simulink model "sphereMPC"  (R2020b)
settings: Solver=ode4  StartTime=0  StopTime=400  FixedStep=0.01  MaxStep=0.01  RelTol=1e-3  EnableMultiTasking=on
values from neighbouring files (symbols this model uses):
  simu = simulationClass()    [plotFreqDep.m]    (also in wecSimInputFile.m)
undefined symbols (not defined in the file or in its folder): body, controller, geometry, hydroData, pto
libraries: WECSim_Lib_Frames x1, WECSim_Lib_Body_Elements x1, simulink x1, WECSim_Lib_PTOs x1
settings Model: Creator=mlawson  LastModifiedBy=akeeste
settings SolverCC: ZeroCrossControl=DisableAll  AlgebraicLoopSolver=LineSearch  AutoInsertRateTranBlk=on
settings DataIOCC: SaveFormat=Array  SaveOutput=off  SaveTime=off  ReturnWorkspaceOutputs=off
settings OptimizationCC: LifeSpan=inf  SimCompilerOptimization=on
settings DebuggingCC: MergeDetectMultiDrivingBlocksExec=none  SolverPrmCheckMsg=warning  AllowSymbolicDim=off  StateNameClashWarn=warning  SFUnexpectedBacktrackingDiag=warning  SFNoUnconditionalDefaultTransitionDiag=warning  SFExecutionAtInitializationDiag=none  ArithmeticOperatorsInVariantConditions=warning
settings HardwareCC: ProdBitPerPointer=32  ProdBitPerSizeT=32  ProdBitPerPtrDiffT=32  ProdLargestAtomicFloat=None  ProdIntDivRoundTo=Undefined  ProdEndianess=Unspecified  ProdWordSize=32  ProdHWDeviceType=32-bit Generic
settings ModelReferenceCC: PropagateVarSize=Only when enabling  PropagateSignalLabelsOutOfModel=off
settings SFSimCC: SimUseLocalCustomCode=off  CustomCodeUndefinedFunction=UseInterfaceOnly
settings RTWCC: RTWUseLocalCustomCode=off
settings CodeAppCC: StateflowObjectComments=on
settings GRTTargetCC: TargetLangStandard=C89/C90 (ANSI)
settings ConfigComp: CovMetricSettings=dw  CovSaveCumulativeToWorkspaceVar=on  CovSaveSingleToWorkspaceVar=on  CovExternalEMLEnable=off  CovSFcnEnable=off
settings SimscapeCC: SimscapeNormalizeSystem=off
settings ConfigurationSet: Description=SimMechanics 2G
settings ExplorerConfigSet: InternalSimMechanicsExplorerSettings="<ExplorerConfiguration><canonicalview>default</canonicalview><TilePanel><TileInfo><Tiles Columns=\"1\" Count=\"1\" Rows=\"1\"><Column Left=\"2\" Weight=\"1\"/><Column Left=\"1335\"/><Row Top=\"2\" Weight=\"1\"/><Row Top=\"911\"/><Tile Height=\"1\" Width=\"1\" X=\"0\" Y=\"0\"/></Tiles></TileInfo><SceneInfo><SceneViewer><BGColor><R>0.60000002384185791</R><G>0.60000002384185791</G><B>0.60000002384185791</B></BGColor><Camera><Position><X>365.37645888990272</X><Y>-369.82486814446582</Y><Z>359.64809521743916</Z></Position><Center><X>-6.7351450971904585</X><Y>2.2867358426280204</Y><Z>-12.463508769654169</Z></Center><Up><X>-0.40824829046386307</X><Y>0.40824829046386307</Y><Z>0.81649658092772615</Z></Up><Left>-57.820127362122818</Left><Right>57.820127362122818</Right><Bottom>-38.308817187253304</Bottom><Top>38.308817187253304</Top></Camera></SceneViewer></SceneInfo></TilePanel></ExplorerConfiguration>"

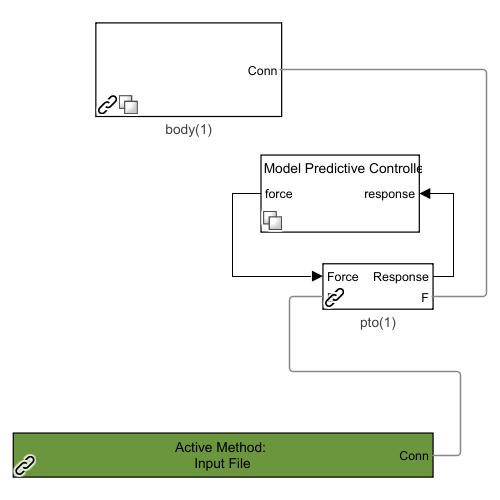
[thumbnail: Simulink's stored preview of the top-level diagram]
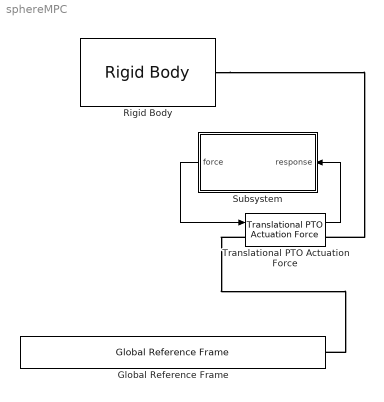
== system sphereMPC ==
  Global Reference Frame : WECSim_Lib_Frames/Global Reference Frame  waves=waves  simu=simu  InputMethod=Input File  InputFile=wecSimInputFile.m  mode=normal  explorer=off  solver=ode4  startTime=0  rampTime=100  endTime=400  dt=0.1  cicEndTime=60  stateSpace=0  WaveClass=regular  height=2.5  period=8  elevationFile=NOT DEFINED  spectrumFile=NOT DEFINED  direction=0  spread=1  spectrumType=NOT DEFINED  phaseSeed=0  option=EqualEnergy
  Rigid Body : WECSim_Lib_Body_Elements/Rigid Body  body=body(1)  h5File=hydroData/*.h5  geometryFile=geometry/*.stl  mass=0  inertia=0 0 0  inertiaProducts=0 0 0  nonHydro=0  nonlinearHydro=0  centerGravity=0 0 0  centerBuoyancy=0 0 0  dof=6  volume=0  QTFs=0  displacement=0 0 0  axis=0 1 0  angle=0  option=0  cd=0 0 0  ca=0 0 0  area=0 0 0  VME=0  rgME=0 0 0  z=0 0 1
  Subsystem : Subsystem  Variant=on  VariantControl=Choice
  Translational PTO Actuation Force : WECSim_Lib_PTOs/Translational PTO Actuation Force  pto=pto(1)  loc="0  0  0"  stiffness=0  damping=0  equilibriumPosition=0  pretension=0  displacement=0 0 0  y=0 1 0  z=0 0 1  upperLimitSpecify=off  upperLimitBound=0  upperLimitTransitionRegionWidth=0  upperLimitStiffness=0  upperLimitDamping=0  lowerLimitSpecify=off  lowerLimitBound=0  lowerLimitTransitionRegionWidth=0  lowerLimitStiffness=0  lowerLimitDamping=0
      settings: AttributesFormatString=%<pto>
  wires:
  Translational PTO Actuation Force/1 -> Subsystem/1(response)
  Subsystem/1(force) -> Translational PTO Actuation Force/1
  connections:
  Rigid Body/RConn1 -- Translational PTO Actuation Force/RConn1
  Translational PTO Actuation Force/LConn1 -- Global Reference Frame/RConn1

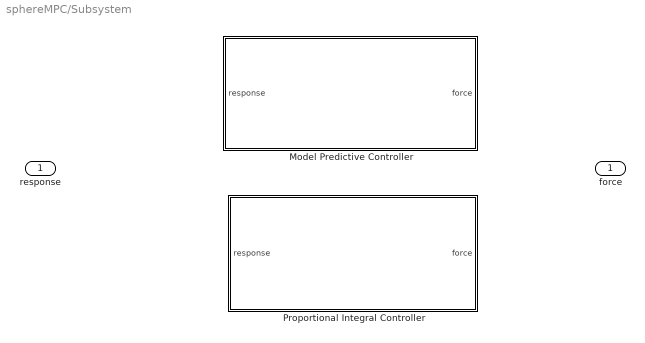
== system sphereMPC/Subsystem ==
  response : Inport
  Model Predictive Controller : Subsystem  VariantControl=controller.MPC == 1
  Proportional Integral Controller : Subsystem  VariantControl=controller.MPC == 0
  force : Outport

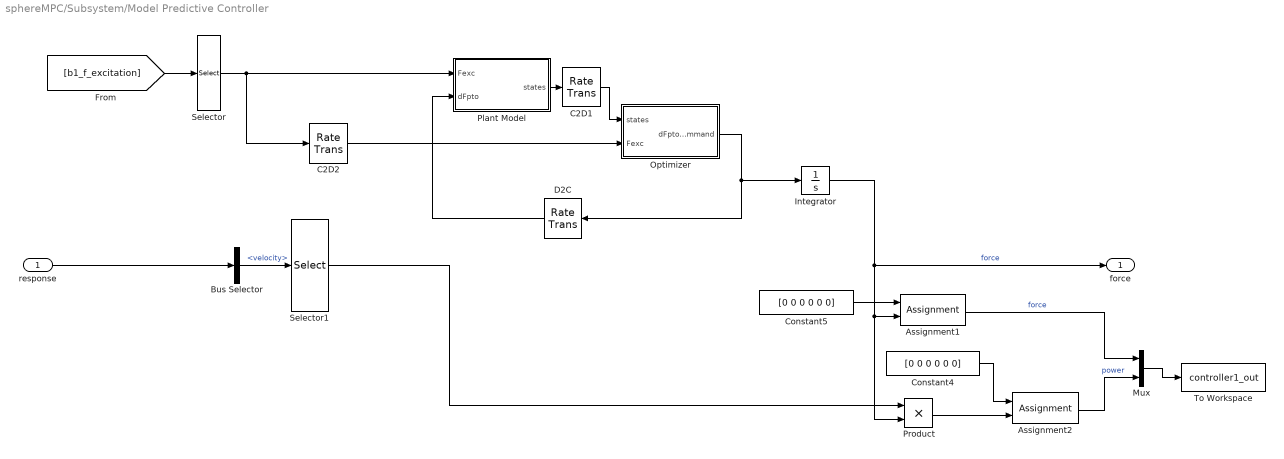
== system sphereMPC/Subsystem/Model Predictive Controller ==
  response : Inport
  Assignment1 : Assignment  IndexOptions=Index vector (dialog)  Indices=3  OutputSizes=1
  Assignment2 : Assignment  IndexOptions=Index vector (dialog)  Indices=3  OutputSizes=1
  Bus Selector : BusSelector  OutputSignals=velocity
  C2D1 : RateTransition  OutPortSampleTime=controller(1).modelPredictiveControl.dt
  C2D2 : RateTransition  OutPortSampleTime=controller(1).modelPredictiveControl.dt
  Constant4 : Constant  Value=[0 0 0 0 0 0]
  Constant5 : Constant  Value=[0 0 0 0 0 0]
  D2C : RateTransition  OutPortSampleTime=simu.dt
  Integrator : Integrator
  Mux : Mux  Inputs=2
  Optimizer : Subsystem
  Plant Model : Subsystem
  Product : Product
  Selector : Selector  InputPortWidth=6  IndexOptions=Index vector (dialog)  Indices=3  OutputSizes=1
  Selector1 : Selector  InputPortWidth=6  IndexOptions=Index vector (dialog)  Indices=3  OutputSizes=1
  To Workspace : ToWorkspace  VariableName=controller1_out  SaveFormat=Structure With Time  SampleTime=simu.dtOut
  force : Outport
  wires:
  Optimizer/1(dFptoCommand) -> D2C/1, Integrator/1
  Assignment1/1 -> Mux/1  "force"
  Integrator/1 -> force/1, Product/2, Assignment1/2  "force"
  [b1_f_excitation] -> Selector/1
  C2D2/1 -> Optimizer/2(Fexc)
  Constant4/1 -> Assignment2/1
  Product/1 -> Assignment2/2
  D2C/1 -> Plant Model/2(dFpto)
  Mux/1 -> To Workspace/1
  Selector1/1 -> Product/1
  Selector/1 -> Plant Model/1(Fexc), C2D2/1
  Constant5/1 -> Assignment1/1
  Plant Model/1(states) -> C2D1/1
  C2D1/1 -> Optimizer/1(states)
  Bus Selector/1 -> Selector1/1  "<velocity>"
  Assignment2/1 -> Mux/2  "power"
  response/1 -> Bus Selector/1

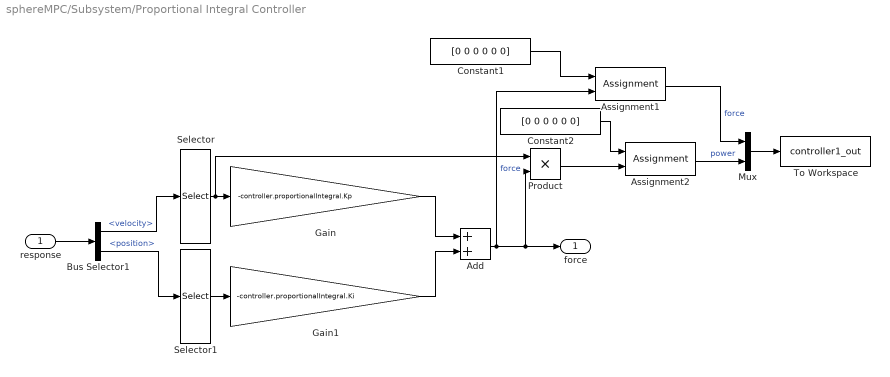
== system sphereMPC/Subsystem/Proportional Integral Controller ==
  response : Inport
  Add : Sum
  Assignment1 : Assignment  IndexOptions=Index vector (dialog)  Indices=3  OutputSizes=1
  Assignment2 : Assignment  IndexOptions=Index vector (dialog)  Indices=3  OutputSizes=1
  Bus Selector1 : BusSelector  OutputSignals=velocity,position
  Constant1 : Constant  Value=[0 0 0 0 0 0]
  Constant2 : Constant  Value=[0 0 0 0 0 0]
  Gain : Gain  Gain=-controller.proportionalIntegral.Kp
  Gain1 : Gain  Gain=-controller.proportionalIntegral.Ki
  Mux : Mux  Inputs=2
  Product : Product
  Selector : Selector  InputPortWidth=6  IndexOptions=Index vector (dialog)  Indices=3  OutputSizes=1
  Selector1 : Selector  InputPortWidth=6  IndexOptions=Index vector (dialog)  Indices=3  OutputSizes=1
  To Workspace : ToWorkspace  VariableName=controller1_out  SaveFormat=Structure With Time  SampleTime=simu.dtOut
  force : Outport
  wires:
  Selector1/1 -> Gain1/1
  Selector/1 -> Gain/1, Product/1
  Bus Selector1/1 -> Selector/1  "<velocity>"
  Constant2/1 -> Assignment2/1
  Product/1 -> Assignment2/2
  Assignment1/1 -> Mux/1  "force"
  Assignment2/1 -> Mux/2  "power"
  Constant1/1 -> Assignment1/1
  Mux/1 -> To Workspace/1
  Bus Selector1/2 -> Selector1/1  "<position>"
  response/1 -> Bus Selector1/1
  Gain/1 -> Add/1
  Add/1 -> Assignment1/2, Product/2, force/1  "force"
  Gain1/1 -> Add/2

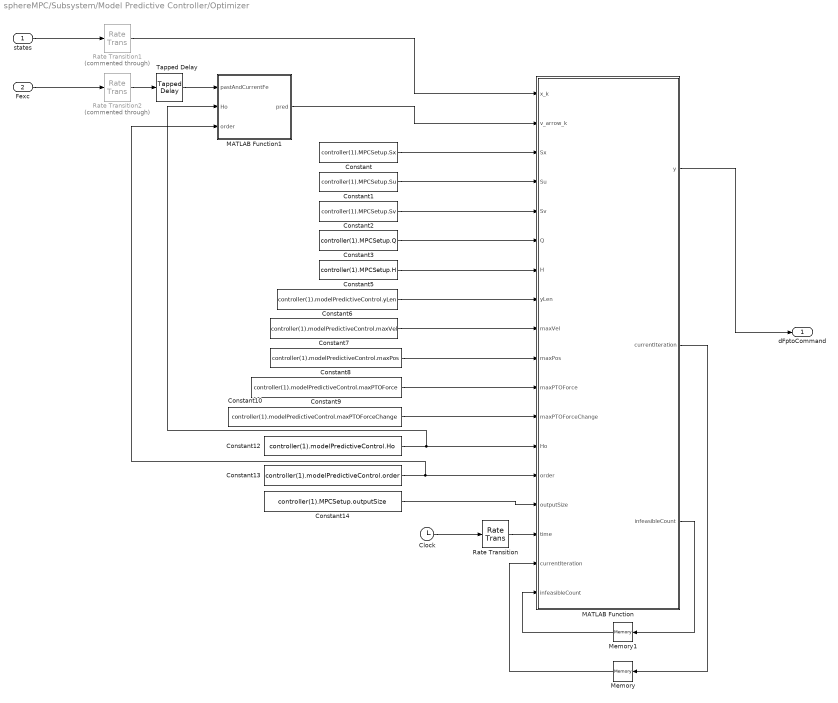
== system sphereMPC/Subsystem/Model Predictive Controller/Optimizer ==
  states : Inport
  Fexc : Inport  Port=2
  Clock : Clock
  Constant : Constant  Value=controller(1).MPCSetup.Sx
  Constant1 : Constant  Value=controller(1).MPCSetup.Su
  Constant10 : Constant  Value=controller(1).modelPredictiveControl.maxPTOForceChange
  Constant12 : Constant  Value=controller(1).modelPredictiveControl.Ho
  Constant13 : Constant  Value=controller(1).modelPredictiveControl.order
  Constant14 : Constant  Value=controller(1).MPCSetup.outputSize
  Constant2 : Constant  Value=controller(1).MPCSetup.Sv
  Constant3 : Constant  Value=controller(1).MPCSetup.Q
  Constant5 : Constant  Value=controller(1).MPCSetup.H
  Constant6 : Constant  Value=controller(1).modelPredictiveControl.yLen
  Constant7 : Constant  Value=controller(1).modelPredictiveControl.maxVel
  Constant8 : Constant  Value=controller(1).modelPredictiveControl.maxPos
  Constant9 : Constant  Value=controller(1).modelPredictiveControl.maxPTOForce
  MATLAB Function : MATLAB Function  TreatAsAtomicUnit=on  SystemSampleTime=controller(1).modelPredictiveControl.dt
  MATLAB Function1 : MATLAB Function  TreatAsAtomicUnit=on
  Memory : Memory
  Memory1 : Memory
  Rate Transition : RateTransition
  Rate Transition1 : RateTransition  Commented=through  OutPortSampleTime=controller(1).modelPredictiveControl.dt
  Rate Transition2 : RateTransition  Commented=through  OutPortSampleTime=controller(1).modelPredictiveControl.dt
  Tapped Delay : simulink/Discrete/Tapped Delay  vinit=0  samptime=-1  NumDelays=controller(1).modelPredictiveControl.Ho + controller(1).modelPredictiveControl.order  DelayOrder=Oldest  includeCurrent=on
  dFptoCommand : Outport
  wires:
  Tapped Delay/1 -> MATLAB Function1/1(pastAndCurrentFe)
  Fexc/1 -> Rate Transition2/1
  Rate Transition2/1 -> Tapped Delay/1
  states/1 -> Rate Transition1/1
  Constant/1 -> MATLAB Function/3(Sx)
  Constant2/1 -> MATLAB Function/5(Sv)
  Constant3/1 -> MATLAB Function/6(Q)
  Constant5/1 -> MATLAB Function/7(H)
  Constant6/1 -> MATLAB Function/8(yLen)
  Constant7/1 -> MATLAB Function/9(maxVel)
  Constant8/1 -> MATLAB Function/10(maxPos)
  Constant9/1 -> MATLAB Function/11(maxPTOForce)
  Constant10/1 -> MATLAB Function/12(maxPTOForceChange)
  Constant12/1 -> MATLAB Function1/2(Ho), MATLAB Function/13(Ho)
  Constant13/1 -> MATLAB Function1/3(order), MATLAB Function/14(order)
  Constant14/1 -> MATLAB Function/15(outputSize)
  MATLAB Function/1(y) -> dFptoCommand/1
  Constant1/1 -> MATLAB Function/4(Su)
  MATLAB Function1/1(pred) -> MATLAB Function/2(v_arrow_k)
  Rate Transition1/1 -> MATLAB Function/1(x_k)
  MATLAB Function/2(currentIteration) -> Memory/1
  Memory/1 -> MATLAB Function/17("currentIteration ")
  Clock/1 -> Rate Transition/1
  Rate Transition/1 -> MATLAB Function/16(time)
  MATLAB Function/3(infeasibleCount) -> Memory1/1
  Memory1/1 -> MATLAB Function/18("infeasibleCount ")

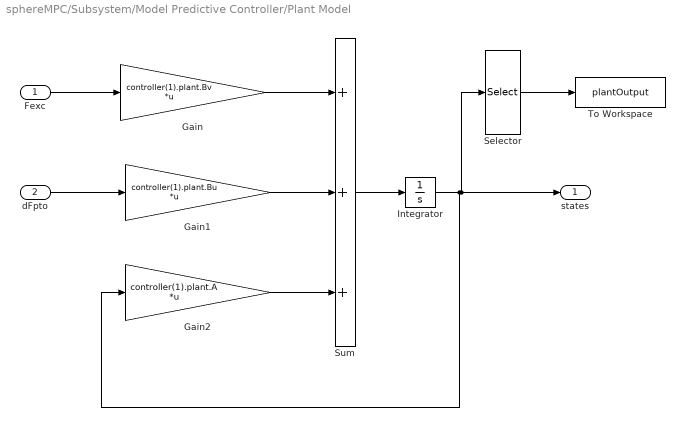
== system sphereMPC/Subsystem/Model Predictive Controller/Plant Model ==
  Fexc : Inport
  dFpto : Inport  Port=2
  Gain : Gain  Gain=controller(1).plant.Bv  Multiplication=Matrix(K*u)
  Gain1 : Gain  Gain=controller(1).plant.Bu  Multiplication=Matrix(K*u)
  Gain2 : Gain  Gain=controller(1).plant.A  Multiplication=Matrix(K*u)
  Integrator : Integrator
  Selector : Selector  InputPortWidth=9  IndexOptions=Index vector (dialog)  Indices=[1 2 9]  OutputSizes=1
  Sum : Sum  Inputs=+++
  To Workspace : ToWorkspace  VariableName=plantOutput  SaveFormat=Timeseries  SampleTime=-1
  states : Outport
  wires:
  Selector/1 -> To Workspace/1
  Integrator/1 -> Gain2/1, Selector/1, states/1
  Sum/1 -> Integrator/1
  Gain2/1 -> Sum/3
  Gain1/1 -> Sum/2
  Gain/1 -> Sum/1
  dFpto/1 -> Gain1/1
  Fexc/1 -> Gain/1

== matlab function sphereMPC/Subsystem/Model Predictive Controller/Optimizer/MATLAB Function ==
  data: x_k input; y output size=1; v_arrow_k input size=[HpInk+1,1]; Sx input; Su input; Sv input; Q input; H input; yLen input; maxVel input; maxPos input; maxPTOForce input; maxPTOForceChange input; Ho input; order input; outputSize input; time input; currentIteration input size=1; infeasibleCount input size=1; currentIteration output; infeasibleCount output; HpInk parameter size=1
function [y, currentIteration, infeasibleCount]  = mpcFcn(x_k, v_arrow_k, Sx, Su, Sv, Q, H, yLen, maxVel, maxPos, maxPTOForce, maxPTOForceChange, Ho, order, outputSize, time, currentIteration, infeasibleCount,  HpInk)

coder.extrinsic('mpcFcn')

y = 0;

[y, currentIteration, infeasibleCount] = mpcFcn(x_k, v_arrow_k, Sx, Su, Sv, Q, HpInk, H, yLen, maxVel, maxPos, maxPTOForce, maxPTOForceChange, Ho, order, outputSize, currentIteration, time, infeasibleCount);

== matlab function sphereMPC/Subsystem/Model Predictive Controller/Optimizer/MATLAB Function1 ==
  data: pastAndCurrentFe input; pred output size=[HpInk+1,1]; Ho input size=1; order input size=1; HpInk parameter size=1
function pred = fexcPrediction(pastAndCurrentFe, Ho, order, HpInk)

coder.extrinsic('fexcPrediction')

pred = zeros(HpInk+1,1);

pred = fexcPrediction(pastAndCurrentFe, HpInk, Ho, order);
